simulink library "uplink_labels_lib"  (Simulink 7.2)
settings: Solver=ode45  SolverMode=SingleTasking  StartTime=0.0  StopTime=10.0  RelTol=1e-3
undefined symbols (not defined in the file or in its folder): Timestep
libraries: simulink x1
settings Model: Creator=cbuttril  LastModifiedBy=cbuttril

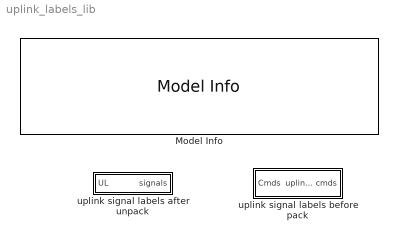
== system uplink_labels_lib ==
  Model Info : simulink/Model-Wide Utilities/Model Info  SystemSampleTime=-1  InitialBlockCM=None  BlockCM=None  Frame=on  DisplayStringWithTags=|  HorizontalTextAlignment=Center  LeftAlignmentValue=0.5  SourceBlockDiagram=uplink_labels_lib  TagMaxNumber=20
      | Developed using Matlab Release 2007a
      | 
      | SVN:%<ModelVersion>
      | Last modifed by %<LastModifiedBy> on %<LastModificationDate>
  uplink signal labels after unpack : Subsystem
  uplink signal labels before pack : Subsystem

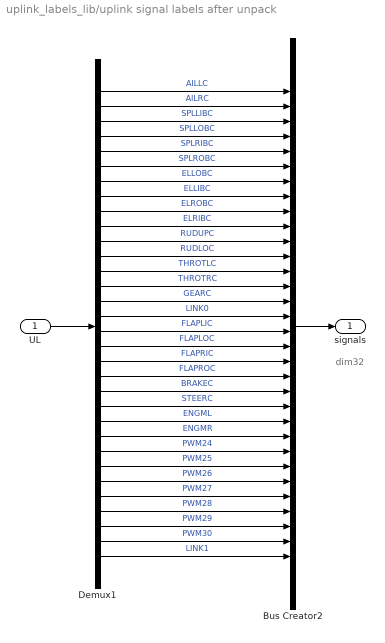
== system uplink_labels_lib/uplink signal labels after unpack ==
  note: dim32
  UL : Inport  OutDataType=sfix(16)  OutScaling=2^0
  Bus Creator2 : BusCreator  Inputs=32
  Demux1 : Demux  Outputs=32
  signals : Outport  PortDimensions=32  OutDataType=sfix(16)  OutScaling=2^0
  wires:
  Demux1/22 -> Bus Creator2/22  "STEERC"
  UL/1 -> Demux1/1
  Demux1/32 -> Bus Creator2/32  "LINK1"
  Demux1/31 -> Bus Creator2/31  "PWM30"
  Demux1/30 -> Bus Creator2/30  "PWM29"
  Demux1/29 -> Bus Creator2/29  "PWM28"
  Demux1/28 -> Bus Creator2/28  "PWM27"
  Demux1/27 -> Bus Creator2/27  "PWM26"
  Demux1/26 -> Bus Creator2/26  "PWM25"
  Demux1/25 -> Bus Creator2/25  "PWM24"
  Demux1/24 -> Bus Creator2/24  "ENGMR"
  Demux1/23 -> Bus Creator2/23  "ENGML"
  Demux1/21 -> Bus Creator2/21  "BRAKEC"
  Demux1/20 -> Bus Creator2/20  "FLAPROC"
  Demux1/19 -> Bus Creator2/19  "FLAPRIC"
  Demux1/18 -> Bus Creator2/18  "FLAPLOC"
  Demux1/17 -> Bus Creator2/17  "FLAPLIC"
  Demux1/16 -> Bus Creator2/16  "LINK0"
  Demux1/15 -> Bus Creator2/15  "GEARC"
  Demux1/14 -> Bus Creator2/14  "THROTRC"
  Demux1/13 -> Bus Creator2/13  "THROTLC"
  Demux1/12 -> Bus Creator2/12  "RUDLOC"
  Demux1/11 -> Bus Creator2/11  "RUDUPC"
  Demux1/10 -> Bus Creator2/10  "ELRIBC"
  Demux1/9 -> Bus Creator2/9  "ELROBC"
  Demux1/8 -> Bus Creator2/8  "ELLIBC"
  Demux1/7 -> Bus Creator2/7  "ELLOBC"
  Demux1/6 -> Bus Creator2/6  "SPLROBC"
  Demux1/5 -> Bus Creator2/5  "SPLRIBC"
  Demux1/4 -> Bus Creator2/4  "SPLLOBC"
  Demux1/3 -> Bus Creator2/3  "SPLLIBC"
  Demux1/2 -> Bus Creator2/2  "AILRC"
  Demux1/1 -> Bus Creator2/1  "AILLC"
  Bus Creator2/1 -> signals/1

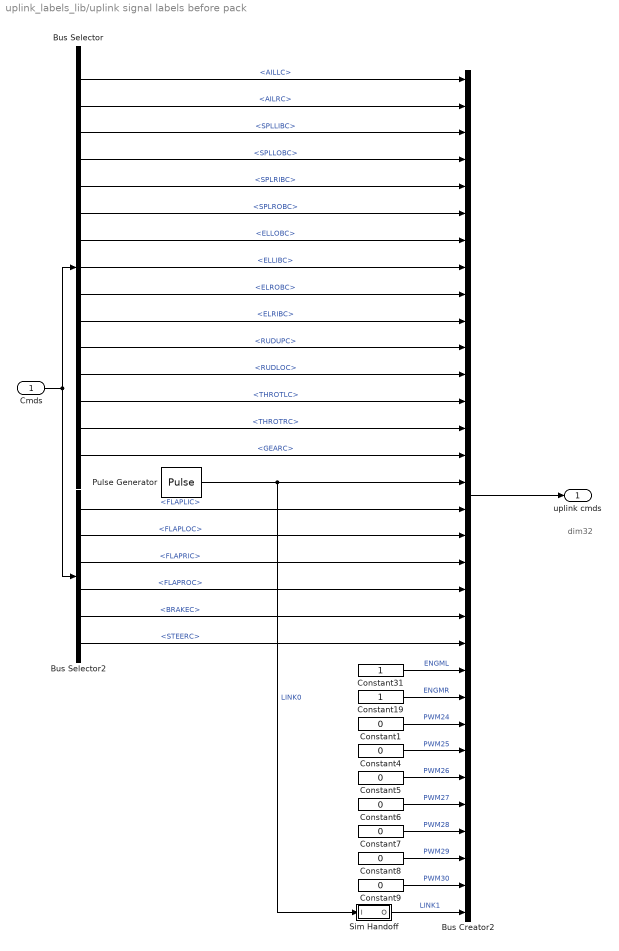
== system uplink_labels_lib/uplink signal labels before pack ==
  note: dim32
  Cmds : Inport  OutDataType=sfix(16)  OutScaling=2^0
  Bus Creator2 : BusCreator  Inputs=32
  Bus Selector : BusSelector  OutputSignals=AILLC,AILRC,SPLLIBC,SPLLOBC,SPLRIBC,SPLROBC,ELLOBC,ELLIBC,ELROBC,ELRIBC,RUDUPC,RUDLOC,THROTLC,THROTRC,GEARC
  Bus Selector2 : BusSelector  OutputSignals=FLAPLIC,FLAPLOC,FLAPRIC,FLAPROC,BRAKEC,STEERC
  Constant{1,4..9} (7 alike) : Constant  Value=0  OutDataType=sfix(16)  OutScaling=2^0
  Constant19 : Constant  OutDataType=sfix(16)  OutScaling=2^0
  Constant31 : Constant  OutDataType=sfix(16)  OutScaling=2^0
  Pulse Generator : DiscretePulseGenerator  Period=12  PulseWidth=6  SampleTime=Timestep
  Sim Handoff : Subsystem
  uplink cmds : Outport  PortDimensions=32  OutDataType=sfix(16)  OutScaling=2^0
  wires:
  Bus Selector2/6 -> Bus Creator2/22  "<STEERC>"
  Bus Selector2/5 -> Bus Creator2/21  "<BRAKEC>"
  Bus Selector/4 -> Bus Creator2/4  "<SPLLOBC>"
  Bus Creator2/1 -> uplink cmds/1
  Constant19/1 -> Bus Creator2/24  "ENGMR"
  Constant31/1 -> Bus Creator2/23  "ENGML"
  Cmds/1 -> Bus Selector/1, Bus Selector2/1
  Bus Selector/1 -> Bus Creator2/1  "<AILLC>"
  Bus Selector/2 -> Bus Creator2/2  "<AILRC>"
  Bus Selector/3 -> Bus Creator2/3  "<SPLLIBC>"
  Bus Selector/5 -> Bus Creator2/5  "<SPLRIBC>"
  Bus Selector/6 -> Bus Creator2/6  "<SPLROBC>"
  Bus Selector/7 -> Bus Creator2/7  "<ELLOBC>"
  Bus Selector/8 -> Bus Creator2/8  "<ELLIBC>"
  Bus Selector/9 -> Bus Creator2/9  "<ELROBC>"
  Bus Selector/10 -> Bus Creator2/10  "<ELRIBC>"
  Bus Selector/11 -> Bus Creator2/11  "<RUDUPC>"
  Bus Selector/12 -> Bus Creator2/12  "<RUDLOC>"
  Bus Selector/13 -> Bus Creator2/13  "<THROTLC>"
  Bus Selector/14 -> Bus Creator2/14  "<THROTRC>"
  Bus Selector/15 -> Bus Creator2/15  "<GEARC>"
  Pulse Generator/1 -> Bus Creator2/16, Sim Handoff/1(I)  "LINK0"
  Bus Selector2/1 -> Bus Creator2/17  "<FLAPLIC>"
  Bus Selector2/2 -> Bus Creator2/18  "<FLAPLOC>"
  Bus Selector2/3 -> Bus Creator2/19  "<FLAPRIC>"
  Bus Selector2/4 -> Bus Creator2/20  "<FLAPROC>"
  Constant1/1 -> Bus Creator2/25  "PWM24"
  Constant4/1 -> Bus Creator2/26  "PWM25"
  Constant5/1 -> Bus Creator2/27  "PWM26"
  Constant6/1 -> Bus Creator2/28  "PWM27"
  Constant7/1 -> Bus Creator2/29  "PWM28"
  Constant8/1 -> Bus Creator2/30  "PWM29"
  Constant9/1 -> Bus Creator2/31  "PWM30"
  Sim Handoff/1(O) -> Bus Creator2/32  "LINK1"

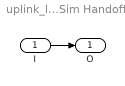
== system uplink_labels_lib/uplink signal labels before pack/Sim Handoff ==
  I : Inport  OutDataType=sfix(16)  OutScaling=2^0
  O : Outport  OutDataType=sfix(16)  OutScaling=2^0
  wires:
  I/1 -> O/1
